simulink model "s1_model_rozszerzony_LQR"  (R2023a)
settings: Solver=ode4  StartTime=0.0  StopTime=end_time  FixedStep=dt  MaxStep=0.001  RelTol=1e-3
values from neighbouring files (symbols this model uses):
  dt = 0.001    [s1_skrypt_rozszerzony_LQR.m]
  E = [1 0 0 0]    [s1_skrypt_rozszerzony_LQR.m]
  F = lqr(A, B, Q, R, N)    [s1_skrypt_rozszerzony_LQR.m]
  IC = [ ... (first row only)    [s1_skrypt_rozszerzony_LQR.m]
  sat = [12, -12]    [s1_skrypt_rozszerzony_LQR.m]
settings Model: Creator=Adam  LastModifiedBy=Adam
settings SolverCC: AlgebraicLoopSolver=TrustRegion
settings DataIOCC: SaveOutput=off  SignalLogging=off  DSMLogging=off
settings DebuggingCC: AlgebraicLoopMsg=none  UnconnectedInputMsg=warning  UnconnectedOutputMsg=warning  UnconnectedLineMsg=warning
settings ModelReferenceCC: EnableRefExpFcnMdlSchedulingChecks=on
settings RTWCC: DLArmComputeVersion=19.05

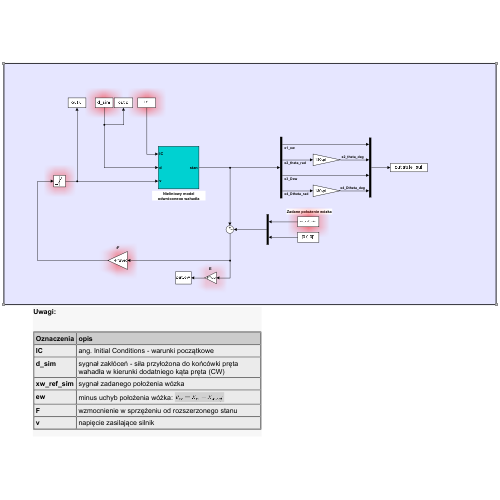
[thumbnail: Simulink's stored preview of the top-level diagram]
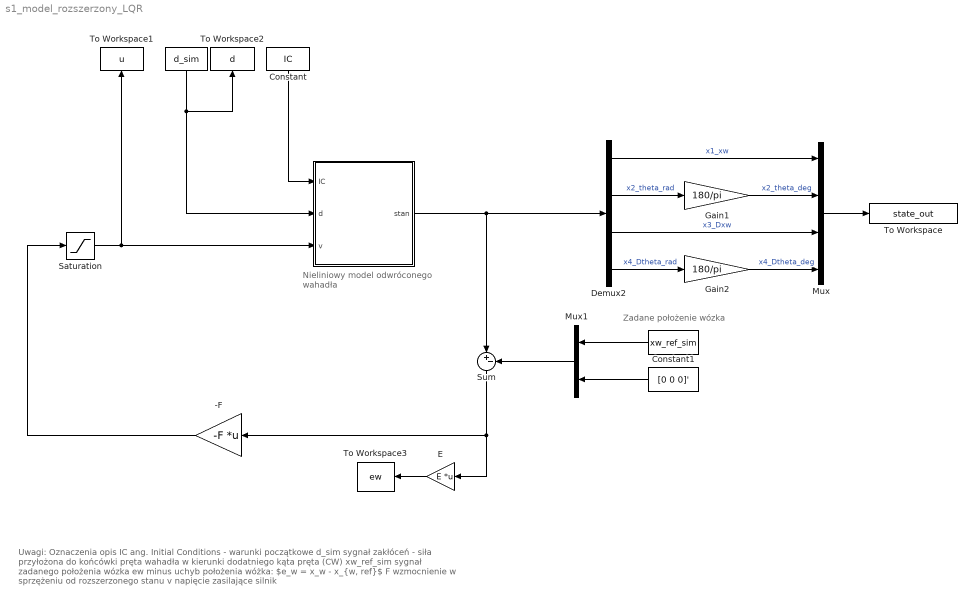
== system s1_model_rozszerzony_LQR ==
  note: Nieliniowy model odwróconego wahadła
  note: Zadane położenie wózka
  note: Uwagi:
      |
      | Oznaczenia
      | opis
      |
      | IC
      | ang. Initial Conditions - warunki początkowe
      |
      | d_sim
      | sygnał zakłóceń - siła przyłożona do końcówki pręta wahadła w kierunki dodatniego kąta pręta (CW)
      |
      | xw_ref_sim
      | sygnał zadanego położenia wózka
      |
      | ew
      | minus uchyb położenia wóżka: $e_w = x_w - x_{w, ref}$
      |
      | F
      | wzmocnienie w sprzężeniu od rozszerzonego stanu
      |
      | v
      | napięcie zasilające silnik
  " " : FromWorkspace  VariableName=xw_ref_sim  SampleTime=dt
  "  " : FromWorkspace  VariableName=d_sim  SampleTime=dt
  "       " : Subsystem  Description=Nonlinear model of inverted pendulum
      mask Display:
      | port_label('output', 1, 'stan');
      | port_label('input', 1, 'IC');
      | port_label('input', 2, 'd');
      | port_label('input', 3, 'v');
  -F : Gain  Gain=-F  Multiplication=Matrix(K*u) (u vector)
  Constant : Constant  Value=IC  VectorParams1D=off
  Constant1 : Constant  Value=[0 0 0]'  VectorParams1D=off
  Demux2 : Demux
  E : Gain  Gain=E  Multiplication=Matrix(K*u) (u vector)
  Gain1 : Gain  Gain=180/pi
  Gain2 : Gain  Gain=180/pi
  Mux : Mux
  Mux1 : Mux  Inputs=2
  Saturation : Saturate  UpperLimit=sat(1)  LowerLimit=sat(2)
  Sum : Sum  Inputs=|+-
  To Workspace : ToWorkspace  VariableName=state_out  SampleTime=-1
  To Workspace1 : ToWorkspace  VariableName=u  SampleTime=-1
  To Workspace2 : ToWorkspace  VariableName=d  SampleTime=-1
  To Workspace3 : ToWorkspace  VariableName=ew  SampleTime=-1
  wires:
  Gain2/1 -> Mux/4  "x4_Dtheta_deg"
  Demux2/4 -> Gain2/1  "x4_Dtheta_rad"
  Demux2/3 -> Mux/3  "x3_Dxw"
  Demux2/2 -> Gain1/1  "x2_theta_rad"
  Demux2/1 -> Mux/1  "x1_xw"
  Gain1/1 -> Mux/2  "x2_theta_deg"
  "       "/1(stan) -> Sum/1, Demux2/1
  Mux/1 -> To Workspace/1
  "  "/1 -> To Workspace2/1, "       "/2(d)
  Constant/1 -> "       "/1(IC)
  " "/1 -> Mux1/1
  Constant1/1 -> Mux1/2
  Mux1/1 -> Sum/2
  Sum/1 -> -F/1, E/1
  E/1 -> To Workspace3/1
  -F/1 -> Saturation/1
  Saturation/1 -> "       "/3(v), To Workspace1/1

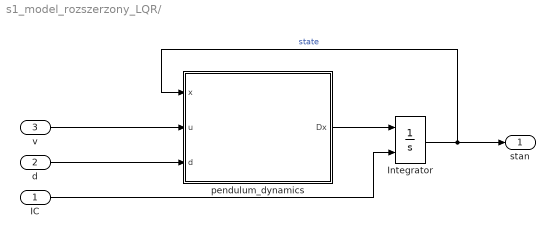
== system s1_model_rozszerzony_LQR/        ==
  IC : Inport
  d : Inport  Port=2
  v : Inport  Port=3
  Integrator : Integrator  InitialConditionSource=external
  pendulum_dynamics : MATLAB Function  TreatAsAtomicUnit=on
  stan : Outport
  wires:
  Integrator/1 -> stan/1, pendulum_dynamics/1(x)  "state"
  v/1 -> pendulum_dynamics/2(u)
  pendulum_dynamics/1(Dx) -> Integrator/1
  IC/1 -> Integrator/2
  d/1 -> pendulum_dynamics/3(d)

== matlab function s1_model_rozszerzony_LQR/       /pendulum_dynamics ==
  data: x input; u input; d input; Dx output; params_lepkie parameter
function Dx = dynamika_wahadla(x, u, d, params_lepkie)
% x : stan
% u : input - napięcie
%
% params scope: "parameters"
%

% State, function input: x = [x Dx theta Dtheta]'
x1 = x(1);
x2 = x(2); 
x3 = x(3);
x4 = x(4);

params_lepkie = num2cell(params_lepkie);
[M, mc, mp, Lp, Lc, g, b, gamma, mr, Mt, L, Jcm, Jt, alpha, beta] = params_lepkie{:};

% Equations for pendulum dynamics
Ff = b*x3;
Fi = alpha*u - beta*x3;
A = d*cos(x2) - Ff + L*mr*x4^2*sin(x2) + Fi;
B = d*Lc + L*g*mr*sin(x2) - gamma*x4;
DEN = Jt*Mt - (L*mr*cos(x2))^2;

ddt_x1 = x3;
ddt_x2 = x4;
ddt_x3 = (Jt*A - L*mr*cos(x2)*B) / DEN;
ddt_x4 = (Mt*B - L*mr*cos(x2)*A) / DEN;

% output (wektor kolumnowy)
Dx = [ddt_x1 ddt_x2 ddt_x3 ddt_x4]';

end
